simulink model "CGMRES"  (R2015a)
settings: Solver=ode45  StartTime=0.0  StopTime=tsim  RelTol=1e-3
values from neighbouring files (symbols this model uses):
  dSamplingPeriod = 0.001    [CGMRES_config.m]
undefined symbols (not defined in the file or in its folder): cgmres, sys
settings Model: Creator=hamada  LastModifiedBy=hamada

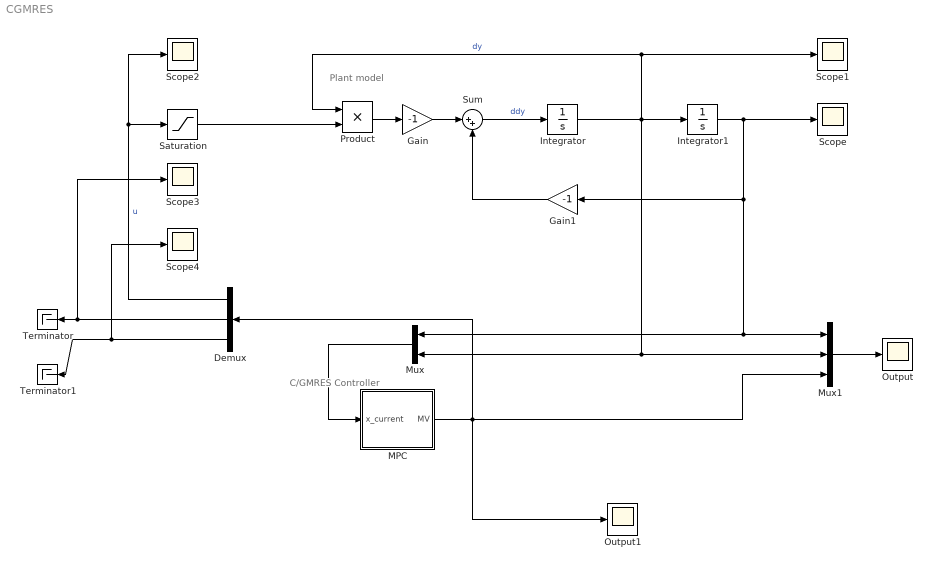
== system CGMRES ==
  note: C/GMRES Controller
  note: Plant model
  Demux : Demux  Outputs=3
  Gain : Gain  Gain=-1
  Gain1 : Gain  Gain=-1
  Integrator : Integrator
  Integrator1 : Integrator  InitialCondition=2
  MPC : MATLAB Function  TreatAsAtomicUnit=on  SystemSampleTime=dSamplingPeriod
  Mux : Mux  Inputs=2
  Mux1 : Mux  Inputs=3
  Output : Scope
      settings: SaveName=Output  SampleInput=on  SampleTime=0.01
  Output1 : Scope
      settings: SaveName=MV  SampleInput=on  SampleTime=dSamplingPeriod
  Product : Product
  Saturation : Saturate  UpperLimit=1  LowerLimit=0
  Scope{,1..4} (5 alike) : Scope
      Scope settings: SaveName=x  SampleInput=on  SampleTime=0.01
      Scope1 settings: SaveName=dx  SampleInput=on  SampleTime=0.01
      Scope2 settings: SaveName=dx1  SampleInput=on  SampleTime=0.01
      Scope3 settings: SaveName=dx2  SampleInput=on  SampleTime=0.01
      Scope4 settings: SaveName=dx3  SampleInput=on  SampleTime=0.01
  Sum : Sum  Inputs=|++
  Terminator : Terminator
  Terminator1 : Terminator
  wires:
  Demux/1 -> Scope2/1, Saturation/1  "u"
  Integrator/1 -> Mux/2, Mux1/2, Scope1/1, Product/1, Integrator1/1  "dy"
  Product/1 -> Gain/1
  Gain1/1 -> Sum/2
  Sum/1 -> Integrator/1  "ddy"
  Gain/1 -> Sum/1
  Integrator1/1 -> Scope/1, Mux/1, Mux1/1, Gain1/1
  Saturation/1 -> Product/2
  MPC/1(MV) -> Output1/1, Demux/1, Mux1/3
  Mux/1 -> MPC/1(x_current)
  Mux1/1 -> Output/1
  Demux/2 -> Scope3/1, Terminator/1
  Demux/3 -> Scope4/1, Terminator1/1

== matlab function CGMRES/MPC ==
  data: x_current input size=2; sys parameter; cgmres parameter; MV output size=3; dSamplingPeriod parameter size=1
function MV = MPC( x_current, sys, cgmres, dSamplingPeriod )
    %#codegen
    persistent flag; % 初回フラグ
    persistent du; % 操作量の変化量（前回値）
    persistent u; % 操作量（前回値）
    persistent T; % 予測区間
    
    if ( isempty( flag ) )
        flag = 0;
    end
    
    if ( isempty( du ) )
        du = zeros( cgmres.len_u * cgmres.dv, 1 );
    end
    
    if ( isempty( u ) )
        u = zeros( cgmres.len_u * cgmres.dv, 1 );
    end
    
    if ( isempty( T ) )
        T = 0;
    end
    
    % 初回のみ操作量の計算方法が異なる
    if ( 0 == flag )
        du = repmat( cgmres.u0, cgmres.dv, 1 );
        u = du;
        flag = 1;
    end 
    
    MV = u(1:cgmres.len_u);
    
    % du = rand( size( du ) ); % 操作量の変化量の初期値は任意に選べるが，前回値を利用すると収束が速い
    du = GMRES( x_current, du, u, T, sys, cgmres );
    u = u + du * dSamplingPeriod;

    T = cgmres.T_outGain * T + cgmres.T_inGain;

end
